simulink model "Dynamics"  (R2022b)
settings: Solver=VariableStepAuto  StartTime=0.0  StopTime=30  FixedStep=1e-3  RelTol=1e-3
model workspace (MAT data in the model file):
  Fd = Simulink.Parameter
  Fd.Value = 0.02
  Fd.DataType = 'double'
  Fd.Complexity = 'real'
  Fd.Dimensions = [1 1]
libraries: simulink x3, vrlib x2, dspindex x2, shared6dof x1, aerolibanim x1, sharedtransform x1
settings Model: Creator=david  LastModifiedBy=david

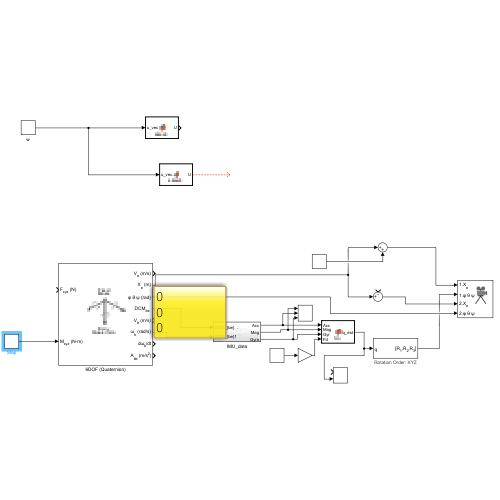
[thumbnail: Simulink's stored preview of the top-level diagram]
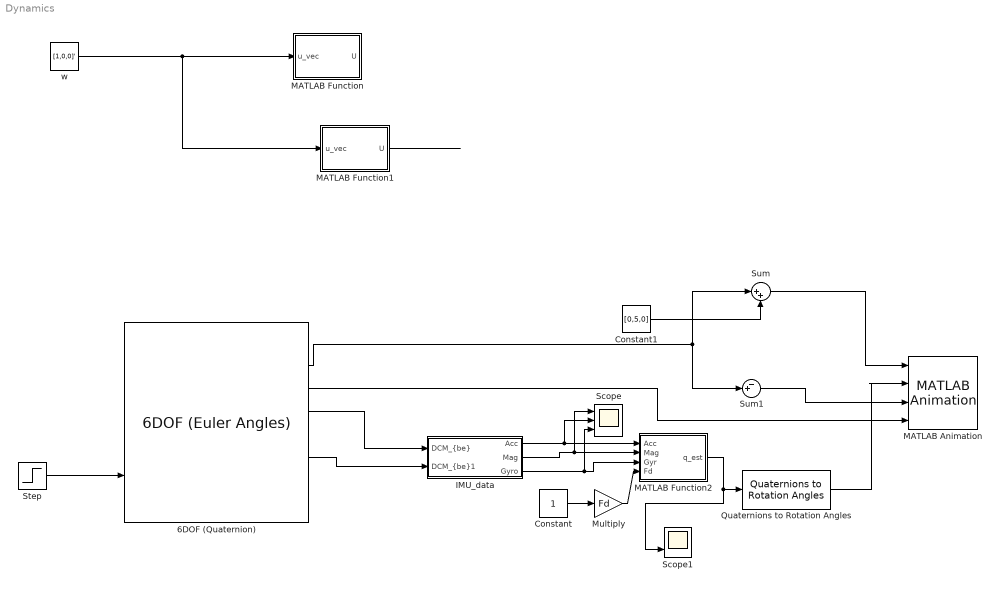
== system Dynamics ==
  6DOF (Quaternion) : shared6dof/6DOF (Euler Angles)  units=Metric (MKS)  mtype=Fixed  rep=Quaternion  xme_0=[0 0 0]  Vm_0=[0 0 0]  eul_0=[0 0 0]  pm_0=[0 0 0]  mass_0=1.0  mass_e=0.5  mass_f=2.0  inertia=eye(3)  inertia_e=eye(3)  inertia_f=2*eye(3)  k_quat=1.0  vre_flag=on  abi_flag=off  aMode=0  xme_statename=''  Vm_statename=''  eul_statename=''  quat_statename=''  pm_statename=''  mass_statename=''
      settings: LibrarySourceBlock=aerolib6dof2/6DOF (Quaternion)
  Constant : Constant
  Constant1 : Constant  Value=[0,5,0]
  IMU_data : Subsystem
  MATLAB Animation : aerolibanim/MATLAB Animation  Tag=Matlab Animation 6 DOF  Vehicles=2  Geometries={'astredwedge.mat','astredwedge.mat'}  BoundingBoxCoordinates=[-50,50,-50,50,-50,50]  CameraOffset=[150,100,-50]  CameraViewAngle=3  SampleTime=0.01  FigurePosition=[7.698000e+02,4.180000e+01,7.664000e+02,7.664000e+02]
  MATLAB Function : MATLAB Function  TreatAsAtomicUnit=on
  MATLAB Function1 : MATLAB Function  TreatAsAtomicUnit=on
  MATLAB Function2 : MATLAB Function  TreatAsAtomicUnit=on  SystemSampleTime=Fd
  Multiply : Gain  Gain=Fd
  Quaternions to Rotation Angles : sharedtransform/Quaternions to Rotation Angles  rotationOrder=XYZ  aMode=aMode
  Scope : Scope  NumInputPorts=3
  Scope1 : Scope  NumInputPorts=2
  Step : Step  Before=[0,0,0.1]'  After=[0,0,0]'  SampleTime=0
  Sum : Sum  Inputs=|++
  Sum1 : Sum  Inputs=-+|
  w : Constant  Value=[1,0,0]'
  wires:
  w/1 -> MATLAB Function1/1(u_vec), MATLAB Function/1(u_vec)
  MATLAB Function1/1(U) -> ?
  Step/1 -> 6DOF (Quaternion)/2
  6DOF (Quaternion)/2 -> Sum1/2, Sum/1
  6DOF (Quaternion)/4 -> IMU_data/1("DCM_{be}")
  6DOF (Quaternion)/6 -> IMU_data/2("DCM_{be}1")
  IMU_data/1(Acc) -> Scope/2, MATLAB Function2/1(Acc)
  IMU_data/3(Gyro) -> Scope/3, MATLAB Function2/3(Gyr)
  Constant/1 -> Multiply/1
  Multiply/1 -> MATLAB Function2/4(Fd)
  Constant1/1 -> Sum/2
  Sum/1 -> MATLAB Animation/1
  Sum1/1 -> MATLAB Animation/3
  MATLAB Function2/1(q_est) -> Scope1/2, Quaternions to Rotation Angles/1
  IMU_data/2(Mag) -> Scope/1, MATLAB Function2/2(Mag)
  Quaternions to Rotation Angles/1 -> MATLAB Animation/2
  6DOF (Quaternion)/3 -> MATLAB Animation/4

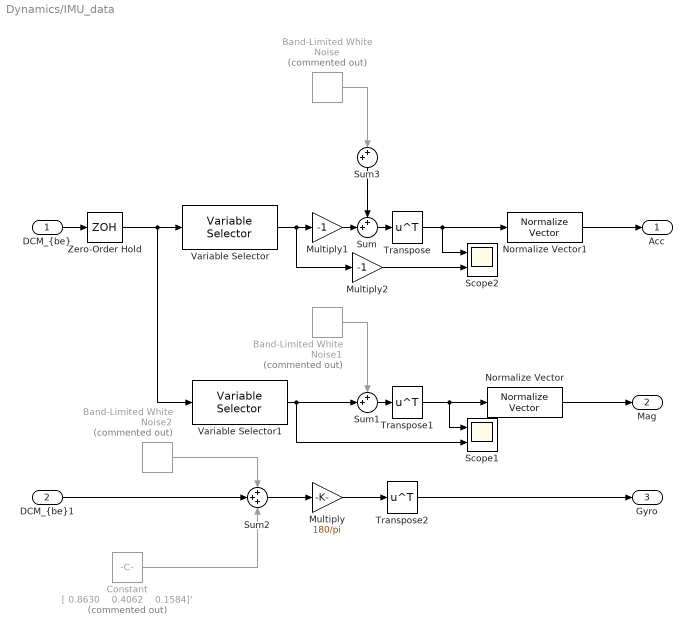
== system Dynamics/IMU_data ==
  "DCM_{be}" : Inport
  "DCM_{be}1" : Inport  Port=2
  Band-Limited White Noise : simulink/Sources/Band-Limited White Noise  Commented=on  Cov="[0.0515    0.0423    0.1177]*1e-4"  Ts=Fd  seed=[23341,23342,23343]  VectorParams1D=off
  Band-Limited White Noise1 : simulink/Sources/Band-Limited White Noise  Commented=on  Cov="[0.2967    0.1789    0.2126]*1e-4"  Ts=Fd  seed=[23344,23345,26343]  VectorParams1D=off
  Band-Limited White Noise2 : simulink/Sources/Band-Limited White Noise  Commented=on  Cov="[0.4540    0.4932    0.3859]*1.0e-07"  Ts=Fd  seed=[21341,22342,33343]  VectorParams1D=off
  Constant : Constant  Commented=on  Value="[ 0.8630    0.4062    0.1584]'"
  Multiply : Gain  Gain=180/pi
  Multiply1 : Gain  Gain=-1
  Multiply2 : Gain  Gain=-1
  Normalize Vector : vrlib/Utilities/Normalize Vector  maxzero=0
  Normalize Vector1 : vrlib/Utilities/Normalize Vector  maxzero=0
  Scope1 : Scope  NumInputPorts=2
  Scope2 : Scope  NumInputPorts=2
  Sum : Sum  Inputs=++|
  Sum1 : Sum  Inputs=++|
  Sum2 : Sum  Inputs=+++
  Sum3 : Sum  Inputs=++|
  Transpose : Math  Operator=transpose
  Transpose1 : Math  Operator=transpose
  Transpose2 : Math  Operator=transpose
  Variable Selector : dspindex/Variable Selector  NumInputs=1  rowsOrCols=Rows  IdxMode=Fixed  Elements=[3]  ZerOneIdxMode=One-based  errmode=Clip Index  FillMode=on  FillValues=0
  Variable Selector1 : dspindex/Variable Selector  NumInputs=1  rowsOrCols=Rows  IdxMode=Fixed  Elements=[1]  ZerOneIdxMode=One-based  errmode=Clip Index  FillMode=on  FillValues=0
  Zero-Order Hold : ZeroOrderHold  SampleTime=Fd
  Acc : Outport
  Mag : Outport  Port=2
  Gyro : Outport  Port=3
  wires:
  Variable Selector/1 -> Multiply2/1, Multiply1/1
  Multiply2/1 -> Scope2/2
  Multiply1/1 -> Sum/2
  Band-Limited White Noise/1 -> Sum3/2
  "DCM_{be}"/1 -> Zero-Order Hold/1
  Zero-Order Hold/1 -> Variable Selector1/1, Variable Selector/1
  Band-Limited White Noise1/1 -> Sum1/1
  Variable Selector1/1 -> Sum1/2, Scope1/2
  "DCM_{be}1"/1 -> Sum2/2
  Sum2/1 -> Multiply/1
  Band-Limited White Noise2/1 -> Sum2/1
  Multiply/1 -> Transpose2/1
  Sum/1 -> Transpose/1
  Transpose/1 -> Scope2/1, Normalize Vector1/1
  Sum1/1 -> Transpose1/1
  Transpose1/1 -> Scope1/1, Normalize Vector/1
  Transpose2/1 -> Gyro/1
  Sum3/1 -> Sum/1
  Constant/1 -> Sum2/3
  Normalize Vector/1 -> Mag/1
  Normalize Vector1/1 -> Acc/1

== matlab function Dynamics/MATLAB Function1 ==
  data: u_vec input; U output
function U = skew4(u_vec)
U = [        0, u_vec(3),-u_vec(2), u_vec(1);
     -u_vec(3),        0, u_vec(1), u_vec(2);
      u_vec(2),-u_vec(1),        0, u_vec(3);
     -u_vec(1),-u_vec(2),-u_vec(3),        0];

== matlab function Dynamics/MATLAB Function ==
  data: u_vec input; U output
function U = skew3(u_vec)
U = [cross([1,0,0]',u_vec),cross([0,1,0]',u_vec),cross([0,0,1]',u_vec)];

== matlab function Dynamics/MATLAB Function2 ==
  data: Acc input; Mag input; Gyr input; q_est output; Fd input
function q_est = fcn(Acc,Mag,Gyr,Fd)
persistent q % q1,q2,q3,q4 with q4 as double
persistent x
persistent P
% Initialization
if isempty(q)
    q = [0,0,0,1]';
end
if isempty(x)
    x = [0,0,0,0,0,0]';
end
if isempty(P)
    P = 10*eye(6,6);
end

% Update state
x = x % No changes in the update step as a is always 0
F = [skew3(Gyr-x(4:6)),-zeros(3,3);
    zeros(3,6)];
G = [-eye(3,3),zeros(3,3);
    zeros(3,3),eye(3,3)];
Q = [1*eye(3,3),zeros(3,3);
   zeros(3,3),1*eye(3,3)];

P = P+Fd*(F*P+P*F'+G*Q*G');
q = (eye(4,4)+Fd/2*skew4(Gyr/180*pi-x(4:6)))*q; % Update the attitude
q = q/norm(q);
A = (q(4)^2-norm(q(1:3))^2)*eye(3,3)+2*q(1:3)*q(1:3)'-2*q(4)*skew3(q(1:3));
% Measurement state
Mag_est = A*[1,0,0]'
Mag
Acc_est = A*[0,0,-1]'
Acc
Ha = [skew3(Acc_est); skew3(Mag_est)];
H = [Ha,zeros(6,3)];

R = [0.01*[1.0000    0.0202   -0.1175
    0.0202    1.0000   -0.0941
   -0.1175   -0.0941    1.0000],zeros(3,3);
zeros(3,3),0.01*eye(3,3)];
K = P*H'/(H*P*H'+R)
innovation = [Acc;Mag]-[Acc_est;Mag_est]
x = x + K*(innovation)
P = P - K*H*P
%Reset state
q_err = [x(1:3)/2; 1-(norm(x(1:3))^2)/8]
q = (skew4(q_err(1:3))+eye(4,4)*q_err(4))*q;
x(1:3) = zeros(3,1);

q_est = [q(4);-q(1:3)]
